simulink model "MMC_phase_hackathon_circuit4_HAAS_may1_localrank_b23"  (R2023b)
settings: Solver=FixedStepDiscrete  StartTime=t_init_sim  StopTime=sim_time  FixedStep=Ts  RelTol=1e-3
values from neighbouring files (symbols this model uses):
  a = 1    [param_phase_circuit4_20260216.m]
  C1low1_active = 1    [script_MMC_phase_circuit4_twist_20260216.m]
  C2low1_active = 1    [script_MMC_phase_circuit4_twist_20260216.m]
  C_bus = 4400e-6    (= 0.0044)    [param_phase_circuit4_20260216.m]
  C_M_extra = C_m-twist_high_side_C    [param_phase_circuit4_20260216.m]
  f0 = 50    [param_phase_circuit4_20260216.m]
  feeder_current_lower_rate_limit = -10    [script_MMC_phase_circuit4_twist_20260216.m]
  is6VExternallySupplied = true    [script_MMC_phase_circuit4_twist_20260216.m]
  isFeederJumperOpen = true    [script_MMC_phase_circuit4_twist_20260216.m]
  L_arm = 60e-3    (= 0.06)    [param_phase_circuit4_20260216.m]
  m = 1    [param_phase_circuit4_20260216.m]
  power_losses = false    [script_MMC_phase_circuit4_twist_20260216.m]
  R = 15    [param_phase_circuit4_20260216.m]
  source_V = 0    [script_MMC_phase_circuit4_twist_20260216.m]
  time_charge = 0.1    [script_MMC_phase_circuit4_twist_20260216.m]
  time_decharge = 1.5    [script_MMC_phase_circuit4_twist_20260216.m]
  Ts = 5e-7    (= 5e-07)    [script_MMC_phase_circuit4_twist_20260216.m]
  twist_data_acquisition_delay = 50e-9    (= 5e-08)    [script_MMC_phase_circuit4_twist_20260216.m]
  twist_data_sampling_period = 1/twist_freq_data_sampling    (= 5e-05)    [script_MMC_phase_circuit4_twist_20260216.m]
  VDC = 48    [param_phase_circuit4_20260216.m]
undefined symbols (not defined in the file or in its folder): C_SM, feeder_current, feeder_current_tab, feeder_current_upper_rate_limit, gcbh, sps_rtmsupport, twist_dead_time, twist_freq_switching, twist_high_side_adc_R, twist_high_side_C, twist_high_side_feeder_R, twist_high_side_rC, twist_low_side_adc_R, twist_low_side_C_ceramic, twist_low_side_C_electrolytic, twist_low_side_L, twist_low_side_lC, twist_low_side_rC, twist_low_side_rL, twist_R_VCC
libraries: spsSeriesRLCBranchLib x135, spsTriangleGeneratorLib x60, spsMosfetLib x60, spsCurrentMeasurementLib x43, spsVoltageMeasurementLib x35, spsControlledCurrentSourceLib x30, spsDiodeLib x22, spsIdealSwitchLib x20, spsControlledVoltageSourceLib x1, spsGroundLib x1, spspowerguiLib x1
(part 18 of 18)

== matlab function MMC_phase_hackathon_circuit4_HAAS_may1_localrank_b23/ /Sinus Modulation + Sorting Algorithm/Subsystem2/Subsystem/MATLAB Function3 ==
  data: sm_id input; m_arm input; gate_signal output; i_arm input; Vc_arm input; Vc_prev input; Vc_next input; N input
function gate_signal = hb_sm_local_ctrl_neighbor(sm_id, m_arm, i_arm, Vc_arm, Vc_prev, Vc_next, N)
%#codegen
% =========================================================
% LOCAL SUBMODULE CONTROLLER WITH NEIGHBOR VOLTAGE BALANCING
% =========================================================
% This function generates the gate signal of one submodule.
%
% Inputs:
%   sm_id   : index of the current submodule inside the arm
%   m_arm   : global arm modulation index, between 0 and 1
%   i_arm   : arm current
%   Vc_arm  : vector of all capacitor voltages in the same arm
%   Vc_prev : capacitor voltage of the previous neighbor submodule
%   Vc_next : capacitor voltage of the next neighbor submodule
%   N       : total number of submodules in the arm
%
% Output:
%   gate_signal : continuous duty signal between 0 and 1
%                 0 means bypassed
%                 1 means inserted
%                 between 0 and 1 means PWM fractional insertion
% =========================================================


% =========================================================
% 1. BALANCING PARAMETER
% =========================================================

k_v = double(0.2);   
% Voltage balancing gain.
% It controls how strongly the local submodule corrects its duty cycle
% according to the difference between its capacitor voltage and neighbor voltages.
% Unit is approximately 1/V.
% If k_v is too high, the gate signal becomes unstable or saturated.
% If k_v is too low, balancing becomes slow.


% =========================================================
% 2. LOCAL NEIGHBOR VOLTAGE REFERENCE
% =========================================================

Vref = double(0.5 * (Vc_prev + Vc_next));
% The local reference voltage is calculated from the average of the two neighbors.
% This is a decentralized idea because the submodule does not need all arm voltages.
% It only compares itself with the previous and next submodules.

v_current = double(Vc_arm(sm_id));
% Read the capacitor voltage of the current submodule.
% sm_id selects which submodule is being controlled.


% =========================================================
% 3. LOCAL VOLTAGE BALANCING CORRECTION
% =========================================================

dm = k_v * (Vref - v_current) * double(sign(i_arm));
% dm is the local correction added to the global modulation index m_arm.
%
% If v_current is lower than Vref:
%   Vref - v_current is positive.
%
% If v_current is higher than Vref:
%   Vref - v_current is negative.
%
% sign(i_arm) makes the correction dependent on current direction.
% This is important because capacitor voltage increases or decreases
% depending on whether the submodule is inserted during positive or negative arm current.

m_i = max(0.0, min(double(m_arm) + dm, 1.0));
% Add the local correction dm to the global arm modulation index.
% Then clamp the result between 0 and 1.
%
% m_i is the corrected local modulation index of this submodule.
% The clamp avoids invalid duty cycles below 0 or above 1.


% =========================================================
% 4. DYNAMIC VOLTAGE RANKING
% =========================================================

n_lower = sum(Vc_arm < v_current);
% Count how many submodules have capacitor voltage lower than the current one.
% This gives the relative position of the current submodule in voltage ranking.

n_equal_lt = sum(Vc_arm(1:sm_id-1) == v_current);
% Count equal-voltage submodules that appear before this submodule.
% This is used to break ties when two or more voltages are equal.
% It ensures that every submodule gets a unique rank.

rank = double(n_lower + n_equal_lt + 1);
% Final voltage rank of the current submodule.
%
% rank = 1 means this submodule has the lowest voltage.
% rank = N means this submodule has the highest voltage.


% =========================================================
% 5. CURRENT-DIRECTION-BASED PRIORITY
% =========================================================

if i_arm >= 0
    % When arm current is positive, inserted submodules are usually charged
    % or discharged depending on the half-bridge current convention.
    % In this implementation, low-voltage submodules are given higher priority.
    
    eff_rank = rank;
    % Keep the natural voltage ranking.
    % Lower-voltage submodules are selected first.

else
    % When arm current is negative, the capacitor energy effect is reversed.
    % Therefore, the insertion priority must also be reversed.
    
    eff_rank = double(N) + 1.0 - rank;
    % Reverse the rank.
    % Higher-voltage submodules are selected first when current direction changes.
end


% =========================================================
% 6. NLM FRACTIONAL DUTY BAND
% =========================================================

duty_low = (eff_rank - 1.0) / double(N);
% Each submodule owns one duty interval or band.
%
% Example for N = 4:
%   Submodule priority 1 owns band from 0.00 to 0.25
%   Submodule priority 2 owns band from 0.25 to 0.50
%   Submodule priority 3 owns band from 0.50 to 0.75
%   Submodule priority 4 owns band from 0.75 to 1.00
%
% duty_low is the lower limit of the current submodule duty band.

duty_raw = (m_i - duty_low) * double(N);
% Convert the corrected modulation index m_i into the local duty of this submodule.
%
% If m_i is below this submodule band:
%   duty_raw becomes negative.
%
% If m_i is inside this submodule band:
%   duty_raw is between 0 and 1.
%
% If m_i is above this submodule band:
%   duty_raw is greater than 1.


% =========================================================
% 7. FINAL GATE SIGNAL CLAMPING
% =========================================================

gate_signal = double(min(max(duty_raw, 0.0), 1.0));
% Clamp duty_raw between 0 and 1.
%
% Final meaning:
%   gate_signal = 0
%       The submodule is bypassed.
%
%   gate_signal = 1
%       The submodule is fully inserted.
%
%   0 < gate_signal < 1
%       The submodule is the boundary submodule and should be driven by PWM.
%
% This output is suitable for an external PWM comparator block.

end

== matlab function MMC_phase_hackathon_circuit4_HAAS_may1_localrank_b23/ /Sinus Modulation + Sorting Algorithm/Subsystem2/Subsystem1/MATLAB Function1 ==
  data: Vc_arm input; i input; Vc_prev output; Vc_next output
function [Vc_prev, Vc_next] = get_neighbors(Vc_arm, i)
%#codegen
% Returns the capacitor voltages of the previous and next (circular) neighbors.
% Hardcoded strictly for N = 5 sub-modules per arm.

N = 5; 

% MATHEMATICAL CIRCULAR INDEXING FOR N = 5:
% If i=1 -> idx_prev = 5, idx_next = 2
% If i=5 -> idx_prev = 4, idx_next = 1

idx_prev = mod(i - 2, N) + 1;
idx_next = mod(i, N) + 1;

Vc_prev = Vc_arm(idx_prev);
Vc_next = Vc_arm(idx_next);

end

== matlab function MMC_phase_hackathon_circuit4_HAAS_may1_localrank_b23/ /Sinus Modulation + Sorting Algorithm/Subsystem2/Subsystem1/MATLAB Function3 ==
  data: sm_id input; m_arm input; gate_signal output; i_arm input; Vc_arm input; Vc_prev input; Vc_next input; N input
function gate_signal = hb_sm_local_ctrl_neighbor(sm_id, m_arm, i_arm, Vc_arm, Vc_prev, Vc_next, N)
%#codegen
% =========================================================
% LOCAL SUBMODULE CONTROLLER WITH NEIGHBOR VOLTAGE BALANCING
% =========================================================
% This function generates the gate signal of one submodule.
%
% Inputs:
%   sm_id   : index of the current submodule inside the arm
%   m_arm   : global arm modulation index, between 0 and 1
%   i_arm   : arm current
%   Vc_arm  : vector of all capacitor voltages in the same arm
%   Vc_prev : capacitor voltage of the previous neighbor submodule
%   Vc_next : capacitor voltage of the next neighbor submodule
%   N       : total number of submodules in the arm
%
% Output:
%   gate_signal : continuous duty signal between 0 and 1
%                 0 means bypassed
%                 1 means inserted
%                 between 0 and 1 means PWM fractional insertion
% =========================================================


% =========================================================
% 1. BALANCING PARAMETER
% =========================================================

k_v = double(0.2);   
% Voltage balancing gain.
% It controls how strongly the local submodule corrects its duty cycle
% according to the difference between its capacitor voltage and neighbor voltages.
% Unit is approximately 1/V.
% If k_v is too high, the gate signal becomes unstable or saturated.
% If k_v is too low, balancing becomes slow.


% =========================================================
% 2. LOCAL NEIGHBOR VOLTAGE REFERENCE
% =========================================================

Vref = double(0.5 * (Vc_prev + Vc_next));
% The local reference voltage is calculated from the average of the two neighbors.
% This is a decentralized idea because the submodule does not need all arm voltages.
% It only compares itself with the previous and next submodules.

v_current = double(Vc_arm(sm_id));
% Read the capacitor voltage of the current submodule.
% sm_id selects which submodule is being controlled.


% =========================================================
% 3. LOCAL VOLTAGE BALANCING CORRECTION
% =========================================================

dm = k_v * (Vref - v_current) * double(sign(i_arm));
% dm is the local correction added to the global modulation index m_arm.
%
% If v_current is lower than Vref:
%   Vref - v_current is positive.
%
% If v_current is higher than Vref:
%   Vref - v_current is negative.
%
% sign(i_arm) makes the correction dependent on current direction.
% This is important because capacitor voltage increases or decreases
% depending on whether the submodule is inserted during positive or negative arm current.

m_i = max(0.0, min(double(m_arm) + dm, 1.0));
% Add the local correction dm to the global arm modulation index.
% Then clamp the result between 0 and 1.
%
% m_i is the corrected local modulation index of this submodule.
% The clamp avoids invalid duty cycles below 0 or above 1.


% =========================================================
% 4. DYNAMIC VOLTAGE RANKING
% =========================================================

n_lower = sum(Vc_arm < v_current);
% Count how many submodules have capacitor voltage lower than the current one.
% This gives the relative position of the current submodule in voltage ranking.

n_equal_lt = sum(Vc_arm(1:sm_id-1) == v_current);
% Count equal-voltage submodules that appear before this submodule.
% This is used to break ties when two or more voltages are equal.
% It ensures that every submodule gets a unique rank.

rank = double(n_lower + n_equal_lt + 1);
% Final voltage rank of the current submodule.
%
% rank = 1 means this submodule has the lowest voltage.
% rank = N means this submodule has the highest voltage.


% =========================================================
% 5. CURRENT-DIRECTION-BASED PRIORITY
% =========================================================

if i_arm >= 0
    % When arm current is positive, inserted submodules are usually charged
    % or discharged depending on the half-bridge current convention.
    % In this implementation, low-voltage submodules are given higher priority.
    
    eff_rank = rank;
    % Keep the natural voltage ranking.
    % Lower-voltage submodules are selected first.

else
    % When arm current is negative, the capacitor energy effect is reversed.
    % Therefore, the insertion priority must also be reversed.
    
    eff_rank = double(N) + 1.0 - rank;
    % Reverse the rank.
    % Higher-voltage submodules are selected first when current direction changes.
end


% =========================================================
% 6. NLM FRACTIONAL DUTY BAND
% =========================================================

duty_low = (eff_rank - 1.0) / double(N);
% Each submodule owns one duty interval or band.
%
% Example for N = 4:
%   Submodule priority 1 owns band from 0.00 to 0.25
%   Submodule priority 2 owns band from 0.25 to 0.50
%   Submodule priority 3 owns band from 0.50 to 0.75
%   Submodule priority 4 owns band from 0.75 to 1.00
%
% duty_low is the lower limit of the current submodule duty band.

duty_raw = (m_i - duty_low) * double(N);
% Convert the corrected modulation index m_i into the local duty of this submodule.
%
% If m_i is below this submodule band:
%   duty_raw becomes negative.
%
% If m_i is inside this submodule band:
%   duty_raw is between 0 and 1.
%
% If m_i is above this submodule band:
%   duty_raw is greater than 1.


% =========================================================
% 7. FINAL GATE SIGNAL CLAMPING
% =========================================================

gate_signal = double(min(max(duty_raw, 0.0), 1.0));
% Clamp duty_raw between 0 and 1.
%
% Final meaning:
%   gate_signal = 0
%       The submodule is bypassed.
%
%   gate_signal = 1
%       The submodule is fully inserted.
%
%   0 < gate_signal < 1
%       The submodule is the boundary submodule and should be driven by PWM.
%
% This output is suitable for an external PWM comparator block.

end

== matlab function MMC_phase_hackathon_circuit4_HAAS_may1_localrank_b23/ /Sinus Modulation + Sorting Algorithm/Subsystem2/Subsystem2/MATLAB Function1 ==
  data: Vc_arm input; i input; Vc_prev output; Vc_next output
function [Vc_prev, Vc_next] = get_neighbors(Vc_arm, i)
%#codegen
% Returns the capacitor voltages of the previous and next (circular) neighbors.
% Hardcoded strictly for N = 5 sub-modules per arm.

N = 5; 

% MATHEMATICAL CIRCULAR INDEXING FOR N = 5:
% If i=1 -> idx_prev = 5, idx_next = 2
% If i=5 -> idx_prev = 4, idx_next = 1

idx_prev = mod(i - 2, N) + 1;
idx_next = mod(i, N) + 1;

Vc_prev = Vc_arm(idx_prev);
Vc_next = Vc_arm(idx_next);

end

== matlab function MMC_phase_hackathon_circuit4_HAAS_may1_localrank_b23/ /Sinus Modulation + Sorting Algorithm/Subsystem2/Subsystem2/MATLAB Function3 ==
  data: sm_id input; m_arm input; gate_signal output; i_arm input; Vc_arm input; Vc_prev input; Vc_next input; N input
function gate_signal = hb_sm_local_ctrl_neighbor(sm_id, m_arm, i_arm, Vc_arm, Vc_prev, Vc_next, N)
%#codegen
% =========================================================
% LOCAL SUBMODULE CONTROLLER WITH NEIGHBOR VOLTAGE BALANCING
% =========================================================
% This function generates the gate signal of one submodule.
%
% Inputs:
%   sm_id   : index of the current submodule inside the arm
%   m_arm   : global arm modulation index, between 0 and 1
%   i_arm   : arm current
%   Vc_arm  : vector of all capacitor voltages in the same arm
%   Vc_prev : capacitor voltage of the previous neighbor submodule
%   Vc_next : capacitor voltage of the next neighbor submodule
%   N       : total number of submodules in the arm
%
% Output:
%   gate_signal : continuous duty signal between 0 and 1
%                 0 means bypassed
%                 1 means inserted
%                 between 0 and 1 means PWM fractional insertion
% =========================================================


% =========================================================
% 1. BALANCING PARAMETER
% =========================================================

k_v = double(0.2);   
% Voltage balancing gain.
% It controls how strongly the local submodule corrects its duty cycle
% according to the difference between its capacitor voltage and neighbor voltages.
% Unit is approximately 1/V.
% If k_v is too high, the gate signal becomes unstable or saturated.
% If k_v is too low, balancing becomes slow.


% =========================================================
% 2. LOCAL NEIGHBOR VOLTAGE REFERENCE
% =========================================================

Vref = double(0.5 * (Vc_prev + Vc_next));
% The local reference voltage is calculated from the average of the two neighbors.
% This is a decentralized idea because the submodule does not need all arm voltages.
% It only compares itself with the previous and next submodules.

v_current = double(Vc_arm(sm_id));
% Read the capacitor voltage of the current submodule.
% sm_id selects which submodule is being controlled.


% =========================================================
% 3. LOCAL VOLTAGE BALANCING CORRECTION
% =========================================================

dm = k_v * (Vref - v_current) * double(sign(i_arm));
% dm is the local correction added to the global modulation index m_arm.
%
% If v_current is lower than Vref:
%   Vref - v_current is positive.
%
% If v_current is higher than Vref:
%   Vref - v_current is negative.
%
% sign(i_arm) makes the correction dependent on current direction.
% This is important because capacitor voltage increases or decreases
% depending on whether the submodule is inserted during positive or negative arm current.

m_i = max(0.0, min(double(m_arm) + dm, 1.0));
% Add the local correction dm to the global arm modulation index.
% Then clamp the result between 0 and 1.
%
% m_i is the corrected local modulation index of this submodule.
% The clamp avoids invalid duty cycles below 0 or above 1.


% =========================================================
% 4. DYNAMIC VOLTAGE RANKING
% =========================================================

n_lower = sum(Vc_arm < v_current);
% Count how many submodules have capacitor voltage lower than the current one.
% This gives the relative position of the current submodule in voltage ranking.

n_equal_lt = sum(Vc_arm(1:sm_id-1) == v_current);
% Count equal-voltage submodules that appear before this submodule.
% This is used to break ties when two or more voltages are equal.
% It ensures that every submodule gets a unique rank.

rank = double(n_lower + n_equal_lt + 1);
% Final voltage rank of the current submodule.
%
% rank = 1 means this submodule has the lowest voltage.
% rank = N means this submodule has the highest voltage.


% =========================================================
% 5. CURRENT-DIRECTION-BASED PRIORITY
% =========================================================

if i_arm >= 0
    % When arm current is positive, inserted submodules are usually charged
    % or discharged depending on the half-bridge current convention.
    % In this implementation, low-voltage submodules are given higher priority.
    
    eff_rank = rank;
    % Keep the natural voltage ranking.
    % Lower-voltage submodules are selected first.

else
    % When arm current is negative, the capacitor energy effect is reversed.
    % Therefore, the insertion priority must also be reversed.
    
    eff_rank = double(N) + 1.0 - rank;
    % Reverse the rank.
    % Higher-voltage submodules are selected first when current direction changes.
end


% =========================================================
% 6. NLM FRACTIONAL DUTY BAND
% =========================================================

duty_low = (eff_rank - 1.0) / double(N);
% Each submodule owns one duty interval or band.
%
% Example for N = 4:
%   Submodule priority 1 owns band from 0.00 to 0.25
%   Submodule priority 2 owns band from 0.25 to 0.50
%   Submodule priority 3 owns band from 0.50 to 0.75
%   Submodule priority 4 owns band from 0.75 to 1.00
%
% duty_low is the lower limit of the current submodule duty band.

duty_raw = (m_i - duty_low) * double(N);
% Convert the corrected modulation index m_i into the local duty of this submodule.
%
% If m_i is below this submodule band:
%   duty_raw becomes negative.
%
% If m_i is inside this submodule band:
%   duty_raw is between 0 and 1.
%
% If m_i is above this submodule band:
%   duty_raw is greater than 1.


% =========================================================
% 7. FINAL GATE SIGNAL CLAMPING
% =========================================================

gate_signal = double(min(max(duty_raw, 0.0), 1.0));
% Clamp duty_raw between 0 and 1.
%
% Final meaning:
%   gate_signal = 0
%       The submodule is bypassed.
%
%   gate_signal = 1
%       The submodule is fully inserted.
%
%   0 < gate_signal < 1
%       The submodule is the boundary submodule and should be driven by PWM.
%
% This output is suitable for an external PWM comparator block.

end

== matlab function MMC_phase_hackathon_circuit4_HAAS_may1_localrank_b23/ /Sinus Modulation + Sorting Algorithm/Subsystem2/Subsystem3/MATLAB Function1 ==
  data: Vc_arm input; i input; Vc_prev output; Vc_next output
function [Vc_prev, Vc_next] = get_neighbors(Vc_arm, i)
%#codegen
% Returns the capacitor voltages of the previous and next (circular) neighbors.
% Hardcoded strictly for N = 5 sub-modules per arm.

N = 5; 

% MATHEMATICAL CIRCULAR INDEXING FOR N = 5:
% If i=1 -> idx_prev = 5, idx_next = 2
% If i=5 -> idx_prev = 4, idx_next = 1

idx_prev = mod(i - 2, N) + 1;
idx_next = mod(i, N) + 1;

Vc_prev = Vc_arm(idx_prev);
Vc_next = Vc_arm(idx_next);

end

== matlab function MMC_phase_hackathon_circuit4_HAAS_may1_localrank_b23/ /Subsystem/Subsystem/Hardware M2/Power losses branch 2/Branch gate loss ==
  data: twist_FET_Pg output
function twist_FET_Pg = powerLossesGate()
    %Twist gate power losses
    twist_freq_switching = 200e3;
    twist_FET_QgH = 31e-9;
    twist_FET_QgL = 31e-9;
    twist_FET_Vgs = 11;

    twist_FET_Pg = (twist_FET_QgH + twist_FET_QgL)*twist_FET_Vgs*twist_freq_switching;
end

== matlab function MMC_phase_hackathon_circuit4_HAAS_may1_localrank_b23/ /Sinus Modulation + Sorting Algorithm/Subsystem2/Subsystem3/MATLAB Function3 ==
  data: sm_id input; m_arm input; gate_signal output; i_arm input; Vc_arm input; Vc_prev input; Vc_next input; N input
function gate_signal = hb_sm_local_ctrl_neighbor(sm_id, m_arm, i_arm, Vc_arm, Vc_prev, Vc_next, N)
%#codegen
% =========================================================
% LOCAL SUBMODULE CONTROLLER WITH NEIGHBOR VOLTAGE BALANCING
% =========================================================
% This function generates the gate signal of one submodule.
%
% Inputs:
%   sm_id   : index of the current submodule inside the arm
%   m_arm   : global arm modulation index, between 0 and 1
%   i_arm   : arm current
%   Vc_arm  : vector of all capacitor voltages in the same arm
%   Vc_prev : capacitor voltage of the previous neighbor submodule
%   Vc_next : capacitor voltage of the next neighbor submodule
%   N       : total number of submodules in the arm
%
% Output:
%   gate_signal : continuous duty signal between 0 and 1
%                 0 means bypassed
%                 1 means inserted
%                 between 0 and 1 means PWM fractional insertion
% =========================================================


% =========================================================
% 1. BALANCING PARAMETER
% =========================================================

k_v = double(0.2);   
% Voltage balancing gain.
% It controls how strongly the local submodule corrects its duty cycle
% according to the difference between its capacitor voltage and neighbor voltages.
% Unit is approximately 1/V.
% If k_v is too high, the gate signal becomes unstable or saturated.
% If k_v is too low, balancing becomes slow.


% =========================================================
% 2. LOCAL NEIGHBOR VOLTAGE REFERENCE
% =========================================================

Vref = double(0.5 * (Vc_prev + Vc_next));
% The local reference voltage is calculated from the average of the two neighbors.
% This is a decentralized idea because the submodule does not need all arm voltages.
% It only compares itself with the previous and next submodules.

v_current = double(Vc_arm(sm_id));
% Read the capacitor voltage of the current submodule.
% sm_id selects which submodule is being controlled.


% =========================================================
% 3. LOCAL VOLTAGE BALANCING CORRECTION
% =========================================================

dm = k_v * (Vref - v_current) * double(sign(i_arm));
% dm is the local correction added to the global modulation index m_arm.
%
% If v_current is lower than Vref:
%   Vref - v_current is positive.
%
% If v_current is higher than Vref:
%   Vref - v_current is negative.
%
% sign(i_arm) makes the correction dependent on current direction.
% This is important because capacitor voltage increases or decreases
% depending on whether the submodule is inserted during positive or negative arm current.

m_i = max(0.0, min(double(m_arm) + dm, 1.0));
% Add the local correction dm to the global arm modulation index.
% Then clamp the result between 0 and 1.
%
% m_i is the corrected local modulation index of this submodule.
% The clamp avoids invalid duty cycles below 0 or above 1.


% =========================================================
% 4. DYNAMIC VOLTAGE RANKING
% =========================================================

n_lower = sum(Vc_arm < v_current);
% Count how many submodules have capacitor voltage lower than the current one.
% This gives the relative position of the current submodule in voltage ranking.

n_equal_lt = sum(Vc_arm(1:sm_id-1) == v_current);
% Count equal-voltage submodules that appear before this submodule.
% This is used to break ties when two or more voltages are equal.
% It ensures that every submodule gets a unique rank.

rank = double(n_lower + n_equal_lt + 1);
% Final voltage rank of the current submodule.
%
% rank = 1 means this submodule has the lowest voltage.
% rank = N means this submodule has the highest voltage.


% =========================================================
% 5. CURRENT-DIRECTION-BASED PRIORITY
% =========================================================

if i_arm >= 0
    % When arm current is positive, inserted submodules are usually charged
    % or discharged depending on the half-bridge current convention.
    % In this implementation, low-voltage submodules are given higher priority.
    
    eff_rank = rank;
    % Keep the natural voltage ranking.
    % Lower-voltage submodules are selected first.

else
    % When arm current is negative, the capacitor energy effect is reversed.
    % Therefore, the insertion priority must also be reversed.
    
    eff_rank = double(N) + 1.0 - rank;
    % Reverse the rank.
    % Higher-voltage submodules are selected first when current direction changes.
end


% =========================================================
% 6. NLM FRACTIONAL DUTY BAND
% =========================================================

duty_low = (eff_rank - 1.0) / double(N);
% Each submodule owns one duty interval or band.
%
% Example for N = 4:
%   Submodule priority 1 owns band from 0.00 to 0.25
%   Submodule priority 2 owns band from 0.25 to 0.50
%   Submodule priority 3 owns band from 0.50 to 0.75
%   Submodule priority 4 owns band from 0.75 to 1.00
%
% duty_low is the lower limit of the current submodule duty band.

duty_raw = (m_i - duty_low) * double(N);
% Convert the corrected modulation index m_i into the local duty of this submodule.
%
% If m_i is below this submodule band:
%   duty_raw becomes negative.
%
% If m_i is inside this submodule band:
%   duty_raw is between 0 and 1.
%
% If m_i is above this submodule band:
%   duty_raw is greater than 1.


% =========================================================
% 7. FINAL GATE SIGNAL CLAMPING
% =========================================================

gate_signal = double(min(max(duty_raw, 0.0), 1.0));
% Clamp duty_raw between 0 and 1.
%
% Final meaning:
%   gate_signal = 0
%       The submodule is bypassed.
%
%   gate_signal = 1
%       The submodule is fully inserted.
%
%   0 < gate_signal < 1
%       The submodule is the boundary submodule and should be driven by PWM.
%
% This output is suitable for an external PWM comparator block.

end

== matlab function MMC_phase_hackathon_circuit4_HAAS_may1_localrank_b23/ /Sinus Modulation + Sorting Algorithm/Subsystem2/Subsystem4/MATLAB Function1 ==
  data: Vc_arm input; i input; Vc_prev output; Vc_next output
function [Vc_prev, Vc_next] = get_neighbors(Vc_arm, i)
%#codegen
% Returns the capacitor voltages of the previous and next (circular) neighbors.
% Hardcoded strictly for N = 5 sub-modules per arm.

N = 5; 

% MATHEMATICAL CIRCULAR INDEXING FOR N = 5:
% If i=1 -> idx_prev = 5, idx_next = 2
% If i=5 -> idx_prev = 4, idx_next = 1

idx_prev = mod(i - 2, N) + 1;
idx_next = mod(i, N) + 1;

Vc_prev = Vc_arm(idx_prev);
Vc_next = Vc_arm(idx_next);

end

== matlab function MMC_phase_hackathon_circuit4_HAAS_may1_localrank_b23/ /Sinus Modulation + Sorting Algorithm/Subsystem2/Subsystem4/MATLAB Function3 ==
  data: sm_id input; m_arm input; gate_signal output; i_arm input; Vc_arm input; Vc_prev input; Vc_next input; N input
function gate_signal = hb_sm_local_ctrl_neighbor(sm_id, m_arm, i_arm, Vc_arm, Vc_prev, Vc_next, N)
%#codegen
% =========================================================
% LOCAL SUBMODULE CONTROLLER WITH NEIGHBOR VOLTAGE BALANCING
% =========================================================
% This function generates the gate signal of one submodule.
%
% Inputs:
%   sm_id   : index of the current submodule inside the arm
%   m_arm   : global arm modulation index, between 0 and 1
%   i_arm   : arm current
%   Vc_arm  : vector of all capacitor voltages in the same arm
%   Vc_prev : capacitor voltage of the previous neighbor submodule
%   Vc_next : capacitor voltage of the next neighbor submodule
%   N       : total number of submodules in the arm
%
% Output:
%   gate_signal : continuous duty signal between 0 and 1
%                 0 means bypassed
%                 1 means inserted
%                 between 0 and 1 means PWM fractional insertion
% =========================================================


% =========================================================
% 1. BALANCING PARAMETER
% =========================================================

k_v = double(0.2);   
% Voltage balancing gain.
% It controls how strongly the local submodule corrects its duty cycle
% according to the difference between its capacitor voltage and neighbor voltages.
% Unit is approximately 1/V.
% If k_v is too high, the gate signal becomes unstable or saturated.
% If k_v is too low, balancing becomes slow.


% =========================================================
% 2. LOCAL NEIGHBOR VOLTAGE REFERENCE
% =========================================================

Vref = double(0.5 * (Vc_prev + Vc_next));
% The local reference voltage is calculated from the average of the two neighbors.
% This is a decentralized idea because the submodule does not need all arm voltages.
% It only compares itself with the previous and next submodules.

v_current = double(Vc_arm(sm_id));
% Read the capacitor voltage of the current submodule.
% sm_id selects which submodule is being controlled.


% =========================================================
% 3. LOCAL VOLTAGE BALANCING CORRECTION
% =========================================================

dm = k_v * (Vref - v_current) * double(sign(i_arm));
% dm is the local correction added to the global modulation index m_arm.
%
% If v_current is lower than Vref:
%   Vref - v_current is positive.
%
% If v_current is higher than Vref:
%   Vref - v_current is negative.
%
% sign(i_arm) makes the correction dependent on current direction.
% This is important because capacitor voltage increases or decreases
% depending on whether the submodule is inserted during positive or negative arm current.

m_i = max(0.0, min(double(m_arm) + dm, 1.0));
% Add the local correction dm to the global arm modulation index.
% Then clamp the result between 0 and 1.
%
% m_i is the corrected local modulation index of this submodule.
% The clamp avoids invalid duty cycles below 0 or above 1.


% =========================================================
% 4. DYNAMIC VOLTAGE RANKING
% =========================================================

n_lower = sum(Vc_arm < v_current);
% Count how many submodules have capacitor voltage lower than the current one.
% This gives the relative position of the current submodule in voltage ranking.

n_equal_lt = sum(Vc_arm(1:sm_id-1) == v_current);
% Count equal-voltage submodules that appear before this submodule.
% This is used to break ties when two or more voltages are equal.
% It ensures that every submodule gets a unique rank.

rank = double(n_lower + n_equal_lt + 1);
% Final voltage rank of the current submodule.
%
% rank = 1 means this submodule has the lowest voltage.
% rank = N means this submodule has the highest voltage.


% =========================================================
% 5. CURRENT-DIRECTION-BASED PRIORITY
% =========================================================

if i_arm >= 0
    % When arm current is positive, inserted submodules are usually charged
    % or discharged depending on the half-bridge current convention.
    % In this implementation, low-voltage submodules are given higher priority.
    
    eff_rank = rank;
    % Keep the natural voltage ranking.
    % Lower-voltage submodules are selected first.

else
    % When arm current is negative, the capacitor energy effect is reversed.
    % Therefore, the insertion priority must also be reversed.
    
    eff_rank = double(N) + 1.0 - rank;
    % Reverse the rank.
    % Higher-voltage submodules are selected first when current direction changes.
end


% =========================================================
% 6. NLM FRACTIONAL DUTY BAND
% =========================================================

duty_low = (eff_rank - 1.0) / double(N);
% Each submodule owns one duty interval or band.
%
% Example for N = 4:
%   Submodule priority 1 owns band from 0.00 to 0.25
%   Submodule priority 2 owns band from 0.25 to 0.50
%   Submodule priority 3 owns band from 0.50 to 0.75
%   Submodule priority 4 owns band from 0.75 to 1.00
%
% duty_low is the lower limit of the current submodule duty band.

duty_raw = (m_i - duty_low) * double(N);
% Convert the corrected modulation index m_i into the local duty of this submodule.
%
% If m_i is below this submodule band:
%   duty_raw becomes negative.
%
% If m_i is inside this submodule band:
%   duty_raw is between 0 and 1.
%
% If m_i is above this submodule band:
%   duty_raw is greater than 1.


% =========================================================
% 7. FINAL GATE SIGNAL CLAMPING
% =========================================================

gate_signal = double(min(max(duty_raw, 0.0), 1.0));
% Clamp duty_raw between 0 and 1.
%
% Final meaning:
%   gate_signal = 0
%       The submodule is bypassed.
%
%   gate_signal = 1
%       The submodule is fully inserted.
%
%   0 < gate_signal < 1
%       The submodule is the boundary submodule and should be driven by PWM.
%
% This output is suitable for an external PWM comparator block.

end

== matlab function MMC_phase_hackathon_circuit4_HAAS_may1_localrank_b23/ /Subsystem/Subsystem/Hardware M2/Power losses branch 2/Branch switching loss ==
  data: VHigh input; twist_FET_Psw output; ILow input
function twist_FET_Psw = powerLossesSwitch(VHigh, ILow)
    %Twist switch power losses
    twist_freq_switching = 200e3;
    twist_FET_trise = 17e-9;
    twist_FET_tfall = 9e-9;

    twist_FET_Psw = 1/2*VHigh*ILow*twist_freq_switching*(twist_FET_trise + twist_FET_tfall);
end
